simulink model "ANPC_ThreeLevelSPWM_AoultSwitch1_WangJiang"  (Simulink 7.9)
settings: Solver=ode23tb  StartTime=0.0  StopTime=1  MaxStep=1e-4  MinStep=1e-5  RelTol=1e-3
undefined symbols (not defined in the file or in its folder): D1, Delta
libraries: powerlib x101, powerlib_extras x1, simulink x1
settings Model: Creator=xieleisky  LastModifiedBy=H002220
settings SolverCC: InitialStep=1e-5
settings OptimizationCC: InitFltsAndDblsToZero=on
settings DebuggingCC: SaveWithParameterizedLinksMsg=none  SignalResolutionControl=TryResolveAllWithWarning  MultiTaskDSMMsg=warning  MultiTaskCondExecSysMsg=none  StrictBusMsg=Warning
settings RTWCC: IncludeERTFirstTime=on
settings GRTTargetCC: TargetFcnLib=ansi_tfl_tmw.mat  CombineOutputUpdateFcns=off  GRTInterface=on

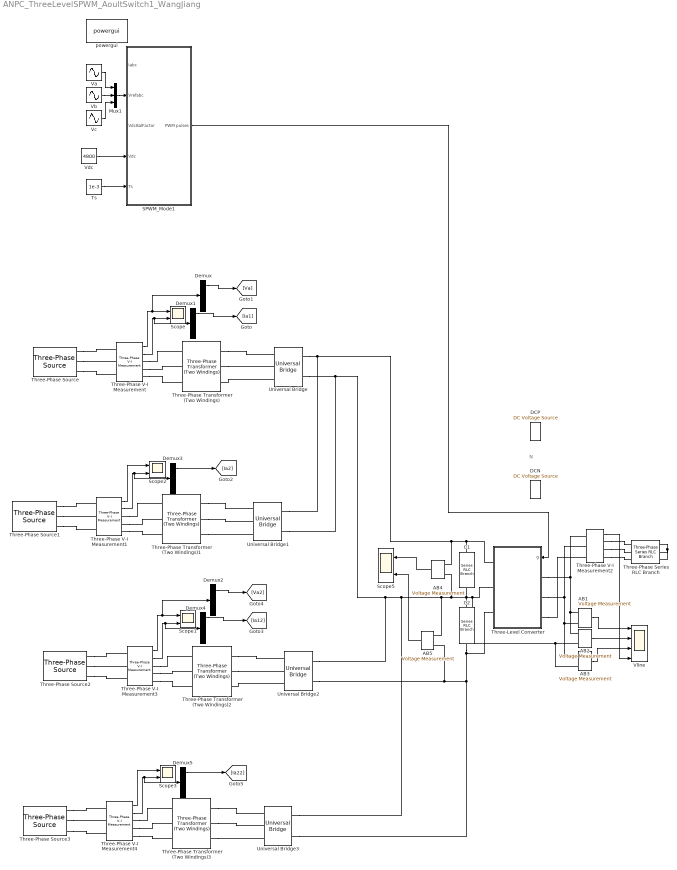
== system ANPC_ThreeLevelSPWM_AoultSwitch1_WangJiang ==
  note: N
  AB{1..5} (5 alike) : powerlib/Measurements/Voltage Measurement  PhasorSimulation=off  OutputType=Complex  PSBequivalent=0
  C1 : powerlib/Elements/Series RLC Branch  LConnTagsString=__new0  RConnTagsString=__new0  BranchType=C  Resistance=1  Inductance=1e-3  SetiL0=off  InitialCurrent=0  Capacitance=8100e-6  Setx0=on  InitialVoltage=2500  Measurements=None
  C2 : powerlib/Elements/Series RLC Branch  LConnTagsString=__new0  RConnTagsString=__new0  BranchType=C  Resistance=1  Inductance=1e-3  SetiL0=off  InitialCurrent=0  Capacitance=8100e-6  Setx0=on  InitialVoltage=2500  Measurements=None
  "DCN " : powerlib/Electrical Sources/DC Voltage Source  Amplitude=300  Measurements=None
  "DCP " : powerlib/Electrical Sources/DC Voltage Source  Amplitude=300  Measurements=None
  Demux{,1..5} (6 alike) : Demux  Outputs=3
  Mux1 : Mux  Inputs=3
  SPWM_Mode1 : Subsystem
  Scope{,1..3,5} (5 alike) : Scope  NumInputPorts=2
      Scope settings: YMin=-5~-5  YMax=5~5
      Scope1 settings: YMin=-5~-5  YMax=5~5  SaveName=ScopeData3
      Scope2 settings: YMin=-5~-5  YMax=5~5  SaveName=ScopeData2
      Scope3 settings: YMin=-5~-5  YMax=5~5  SaveName=ScopeData5
      Scope5 settings: YMin=-5~-5  YMax=5~5  SaveName=ScopeData7
  Three-Level Converter : Subsystem
  Three-Phase Series RLC Branch : powerlib/Elements/Three-Phase Series RLC Branch  LConnTagsString=A|B|C  RConnTagsString=A|B|C  BranchType=RL  Resistance=24.12  Inductance=10.5e-3  Capacitance=1e-6  Measurements=None
  Three-Phase Transformer (Two Windings){,1..3} (4 alike) : powerlib/Elements/Three-Phase Transformer (Two Windings)  Winding1Connection=Delta (D1)  UNITS=pu  NominalPower=[ 1.25e6 , 50 ]  Winding1=[ 25e3 , 0.002 , 0.01 ]  Winding2Connection=Delta (D1)  Winding2=[ 1.8e3 , 0.002 , 0.064 ]  SetSaturation=off  Rm=500  Lm=500  Saturation=[ 0,0 ; 0.0024,1.2 ; 1.0,1.52 ]  Hysteresis=off  DataFile='hysteresis'  SetInitialFlux=off  InitialFluxes=[ 0.8 , -0.8 , 0.7 ]  Measurements=None  MoreParameters=off  BreakLoop=off  DataType=off  TransfoNumber=1
  Three-Phase V-I Measurement{,1,3..4} (4 alike) : powerlib/Measurements/Three-Phase V-I Measurement  VoltageMeasurement=phase-to-phase  SetLabelV=off  LabelV=Vabc  Vpu=off  VpuLL=off  CurrentMeasurement=yes  SetLabelI=off  LabelI=Iabc  Ipu=off  Pbase=100e6  Vbase=500e3  OutputType=Complex  PhasorSimulation=off  PSBequivalent=0
  Three-Phase V-I Measurement2 : powerlib/Measurements/Three-Phase V-I Measurement  VoltageMeasurement=no  SetLabelV=off  LabelV=Vabc  Vpu=off  VpuLL=off  CurrentMeasurement=yes  SetLabelI=off  LabelI=Iabc  Ipu=off  Pbase=100e6  Vbase=500e3  OutputType=Complex  PhasorSimulation=off  PSBequivalent=0
  Three-Phase Source : powerlib/Electrical Sources/Three-Phase Source  Voltage=25e3  PhaseAngle=0  Frequency=50  InternalConnection=Yg  SpecifyImpedance=off  Resistance=1e-5  Inductance=1e-6  ShortCircuitLevel=1e8  BaseVoltage=25e3  XRratio=0.1  BusType=swing  Pref=0  Qref=0  Qmin=-inf  Qmax=inf
  Three-Phase Source1 : powerlib/Electrical Sources/Three-Phase Source  Voltage=25e3  PhaseAngle=15  Frequency=50  InternalConnection=Yg  SpecifyImpedance=off  Resistance=1e-5  Inductance=1e-6  ShortCircuitLevel=1e8  BaseVoltage=25e3  XRratio=0.1  BusType=swing  Pref=0  Qref=0  Qmin=-inf  Qmax=inf
  Three-Phase Source2 : powerlib/Electrical Sources/Three-Phase Source  Voltage=25e3  PhaseAngle=45  Frequency=50  InternalConnection=Yg  SpecifyImpedance=off  Resistance=1e-5  Inductance=1e-6  ShortCircuitLevel=1e8  BaseVoltage=25e3  XRratio=0.1  BusType=swing  Pref=0  Qref=0  Qmin=-inf  Qmax=inf
  Three-Phase Source3 : powerlib/Electrical Sources/Three-Phase Source  Voltage=25e3  PhaseAngle=60  Frequency=50  InternalConnection=Yg  SpecifyImpedance=off  Resistance=1e-5  Inductance=1e-6  ShortCircuitLevel=1e8  BaseVoltage=25e3  XRratio=0.1  BusType=swing  Pref=0  Qref=0  Qmin=-inf  Qmax=inf
  Ts : Constant  Value=1e-3
  Universal Bridge{,1..3} (4 alike) : powerlib/Power Electronics/Universal Bridge  Arms=3  SnubberResistance=1e5  SnubberCapacitance=inf  Device=Diodes  Ron=1e-3  Lon=0  ForwardVoltages="[  0  0  ]"  ForwardVoltage=0.2  GTOparameters=[ 10e-6 , 20e-6 ]  IGBTparameters=[ 1e-6 , 2e-6 ]  Measurements=None  Measurements_2=None  converterType=Rectifier
  Va : Sin  Amplitude=2694  Frequency=100*pi  SampleTime=0
  Vb : Sin  Amplitude=2694  Frequency=100*pi  Phase=-2*pi/3  SampleTime=0
  Vc : Sin  Amplitude=2694  Frequency=100*pi  Phase=2*pi/3  SampleTime=0
  Vdc : Constant  Value=4800
  Vline : Scope  NumInputPorts=4
      settings: TimeRange=0.07315761161915008  YMin=-800~-400~-400~-30  YMax=800~400~400~30  SaveName=A  MaxDataPoints=50000  SampleTime=0.00001
  powergui : powerlib/powergui  SimulationMode=Discrete  SolverType=Tustin  SampleTime=1e-5  frequency=60  SPID=off  DisableSnubberDevices=off  DisableRonSwitches=off  DisableVfSwitches=off  SwTol=0  Interpol=off  DisplayEquations=off  FunctionMessages=off  frequencyindice=0  Pbase=100e6  ErrMax=1e-4  Iterations=50  UnitsV=kV  UnitsW=MW  echomessages=off  HookPort=off  EnableUseOfTLC=off  x0status=blocks  RestoreLinks=warning  ResistiveCurrentMeasurement=off  Frange=[0:2:500]  Ylog=off  Xlog=on  ShowGrid=off  save=off  variable=ZData  structure=ScopeData7  ZoomFFT=off  StartTime=0.2  cycles=1  DisplayStyle=3  fundamental=60  FreqAxis=on  MaxFrequency=3500  frequencyindicesteady=1  RmsSteady=1  display=off  Ts=0  methode=off
  wires:
  Ts/1 -> SPWM_Mode1/5(Ts)
  Vdc/1 -> SPWM_Mode1/4(Vdc)
  AB1/1 -> Vline/1
  AB2/1 -> Vline/2
  AB3/1 -> Vline/3
  Three-Phase V-I Measurement2/1 -> Vline/4
  SPWM_Mode1/1(PWM pulses) -> Three-Level Converter/1(g)
  Mux1/1 -> SPWM_Mode1/2(Vrefabc)
  Vb/1 -> Mux1/2
  Vc/1 -> Mux1/3
  Va/1 -> Mux1/1
  Three-Phase V-I Measurement/2 -> Scope/2, Demux1/1
  Three-Phase V-I Measurement/1 -> Scope/1, Demux/1
  Demux1/1 -> [Ia1]
  Three-Phase V-I Measurement1/2 -> Demux3/1, Scope2/2
  Three-Phase V-I Measurement1/1 -> Scope2/1
  Demux3/1 -> [Ia2]
  Three-Phase V-I Measurement3/2 -> Demux4/1, Scope1/2
  Three-Phase V-I Measurement3/1 -> Demux2/1, Scope1/1
  Demux4/1 -> [Ia12]
  Demux2/1 -> [Va2]
  Three-Phase V-I Measurement4/2 -> Scope3/2, Demux5/1
  Three-Phase V-I Measurement4/1 -> Scope3/1
  Demux5/1 -> [Ia22]
  AB4/1 -> Scope5/1
  AB5/1 -> Scope5/2
  Demux/1 -> [Va]
  connections:
  Three-Level Converter/LConn1 -- AB2/LConn1 -- AB1/LConn1 -- Three-Phase V-I Measurement2/LConn1
  Three-Level Converter/LConn2 -- AB3/LConn1 -- AB1/LConn2 -- Three-Phase V-I Measurement2/LConn2
  Three-Level Converter/LConn3 -- Three-Phase V-I Measurement2/LConn3
  Three-Phase Series RLC Branch/RConn1 -- Three-Phase Series RLC Branch/RConn2 -- Three-Phase Series RLC Branch/RConn3
  Three-Phase V-I Measurement2/RConn1 -- Three-Phase Series RLC Branch/LConn1
  Three-Phase V-I Measurement2/RConn2 -- Three-Phase Series RLC Branch/LConn2
  Three-Phase V-I Measurement2/RConn3 -- Three-Phase Series RLC Branch/LConn3
  Three-Phase V-I Measurement/RConn3 -- Three-Phase Transformer (Two Windings)/LConn3
  Three-Phase Source1/RConn2 -- Three-Phase V-I Measurement1/LConn2
  Three-Phase Source1/RConn3 -- Three-Phase V-I Measurement1/LConn3
  Three-Phase V-I Measurement1/RConn1 -- Three-Phase Transformer (Two Windings)1/LConn1
  Three-Phase Transformer (Two Windings)1/RConn1 -- Universal Bridge1/LConn1
  Three-Phase V-I Measurement1/RConn3 -- Three-Phase Transformer (Two Windings)1/LConn3
  Three-Phase Source/RConn3 -- Three-Phase V-I Measurement/LConn3
  Three-Phase Transformer (Two Windings)/RConn3 -- Universal Bridge/LConn3
  Three-Phase Source1/RConn1 -- Three-Phase V-I Measurement1/LConn1
  Three-Phase V-I Measurement/RConn1 -- Three-Phase Transformer (Two Windings)/LConn1
  Three-Phase Transformer (Two Windings)1/RConn2 -- Universal Bridge1/LConn2
  Three-Phase V-I Measurement/RConn2 -- Three-Phase Transformer (Two Windings)/LConn2
  Three-Phase Transformer (Two Windings)/RConn1 -- Universal Bridge/LConn1
  Three-Phase Source/RConn1 -- Three-Phase V-I Measurement/LConn1
  Three-Phase Source/RConn2 -- Three-Phase V-I Measurement/LConn2
  Three-Phase Transformer (Two Windings)/RConn2 -- Universal Bridge/LConn2
  Three-Phase V-I Measurement1/RConn2 -- Three-Phase Transformer (Two Windings)1/LConn2
  Three-Phase Transformer (Two Windings)1/RConn3 -- Universal Bridge1/LConn3
  Universal Bridge2/RConn2 -- C2/RConn1 -- Three-Level Converter/RConn3 -- Universal Bridge3/RConn2 -- AB5/LConn2
  Universal Bridge/RConn1 -- Universal Bridge1/RConn1 -- Three-Level Converter/RConn1 -- C1/LConn1 -- AB4/LConn1
  C1/RConn1 -- C2/LConn1 -- Three-Level Converter/RConn2 -- AB4/LConn2 -- Universal Bridge/RConn2 -- Universal Bridge1/RConn2 -- Universal Bridge2/RConn1 -- Universal Bridge3/RConn1 -- AB5/LConn1 -- AB2/LConn2 -- AB3/LConn2
  Three-Phase Source2/RConn1 -- Three-Phase V-I Measurement3/LConn1
  Three-Phase Source2/RConn3 -- Three-Phase V-I Measurement3/LConn3
  Three-Phase Transformer (Two Windings)3/RConn1 -- Universal Bridge3/LConn1
  Three-Phase Transformer (Two Windings)3/RConn2 -- Universal Bridge3/LConn2
  Three-Phase Source3/RConn3 -- Three-Phase V-I Measurement4/LConn3
  Three-Phase Source3/RConn2 -- Three-Phase V-I Measurement4/LConn2
  Three-Phase Transformer (Two Windings)2/RConn2 -- Universal Bridge2/LConn2
  Three-Phase Transformer (Two Windings)3/RConn3 -- Universal Bridge3/LConn3
  Three-Phase Source2/RConn2 -- Three-Phase V-I Measurement3/LConn2
  Three-Phase V-I Measurement4/RConn1 -- Three-Phase Transformer (Two Windings)3/LConn1
  Three-Phase V-I Measurement4/RConn2 -- Three-Phase Transformer (Two Windings)3/LConn2
  Three-Phase Transformer (Two Windings)2/RConn1 -- Universal Bridge2/LConn1
  Three-Phase Source3/RConn1 -- Three-Phase V-I Measurement4/LConn1
  Three-Phase V-I Measurement3/RConn1 -- Three-Phase Transformer (Two Windings)2/LConn1
  Three-Phase Transformer (Two Windings)2/RConn3 -- Universal Bridge2/LConn3
  Three-Phase V-I Measurement3/RConn3 -- Three-Phase Transformer (Two Windings)2/LConn3
  Three-Phase V-I Measurement4/RConn3 -- Three-Phase Transformer (Two Windings)3/LConn3
  Three-Phase V-I Measurement3/RConn2 -- Three-Phase Transformer (Two Windings)2/LConn2

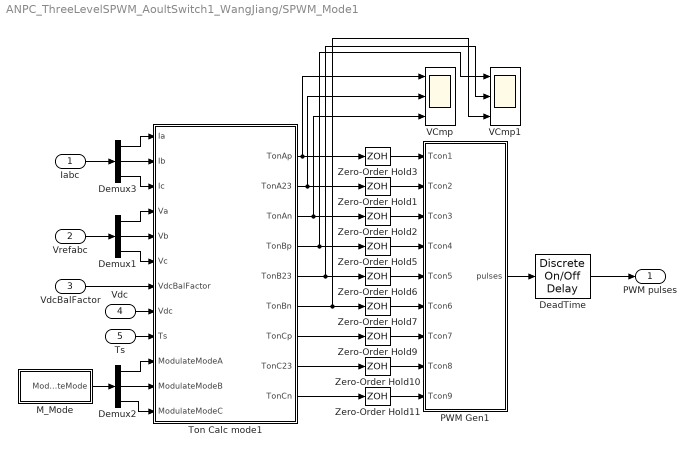
== system ANPC_ThreeLevelSPWM_AoultSwitch1_WangJiang/SPWM_Mode1 ==
  Iabc : Inport
  Vrefabc : Inport  Port=2
  VdcBalFactor : Inport  Port=3
  Vdc : Inport  Port=4
  Ts : Inport  Port=5
  DeadTime : powerlib_extras/Discrete  Control Blocks/Discrete On//Off Delay  type_delay=On delay  delay=20e-6  ic=4e-5  Ts=1e-5
  Demux1 : Demux  Outputs=3
  Demux2 : Demux  Outputs=3
  Demux3 : Demux  Outputs=3
  M_Mode : Subsystem
  PWM Gen1 : Subsystem
  Ton Calc mode1 : MATLAB Function  TreatAsAtomicUnit=on
  VCmp : Scope  NumInputPorts=3
      settings: TimeRange=0.5  YMin=0.00015~0~0.00065  YMax=0.00035~0.001~0.00085  SaveName=A3  MaxDataPoints=50000  SampleTime=0.00001
  VCmp1 : Scope  NumInputPorts=3
      settings: TimeRange=0.05095198250172486  YMin=0~0~0  YMax=0.001~0.001~0.001  SaveName=A1  MaxDataPoints=50000  SampleTime=0.00001
  Zero-Order Hold{1..3,5..7,9..11} (9 alike) : ZeroOrderHold  SampleTime=1/1500
  PWM pulses : Outport
  wires:
  Demux1/2 -> Ton Calc mode1/5(Vb)
  Demux1/3 -> Ton Calc mode1/6(Vc)
  Vdc/1 -> Ton Calc mode1/8(Vdc)
  Ts/1 -> Ton Calc mode1/9(Ts)
  Zero-Order Hold3/1 -> PWM Gen1/1(Tcon1)
  Zero-Order Hold2/1 -> PWM Gen1/3(Tcon3)
  Zero-Order Hold11/1 -> PWM Gen1/9(Tcon9)
  PWM Gen1/1(pulses) -> DeadTime/1
  Zero-Order Hold10/1 -> PWM Gen1/8(Tcon8)
  Zero-Order Hold9/1 -> PWM Gen1/7(Tcon7)
  Zero-Order Hold7/1 -> PWM Gen1/6(Tcon6)
  Zero-Order Hold6/1 -> PWM Gen1/5(Tcon5)
  Zero-Order Hold5/1 -> PWM Gen1/4(Tcon4)
  Zero-Order Hold1/1 -> PWM Gen1/2(Tcon2)
  Ton Calc mode1/1(TonAp) -> VCmp/1, Zero-Order Hold3/1
  Ton Calc mode1/2(TonA23) -> VCmp/2, Zero-Order Hold1/1
  Ton Calc mode1/3(TonAn) -> VCmp/3, Zero-Order Hold2/1
  Ton Calc mode1/4(TonBp) -> VCmp1/1, Zero-Order Hold5/1
  Ton Calc mode1/5(TonB23) -> VCmp1/2, Zero-Order Hold6/1
  Ton Calc mode1/6(TonBn) -> VCmp1/3, Zero-Order Hold7/1
  Ton Calc mode1/7(TonCp) -> Zero-Order Hold9/1
  Ton Calc mode1/8(TonC23) -> Zero-Order Hold10/1
  Ton Calc mode1/9(TonCn) -> Zero-Order Hold11/1
  Demux3/1 -> Ton Calc mode1/1(Ia)
  Demux3/2 -> Ton Calc mode1/2(Ib)
  Demux3/3 -> Ton Calc mode1/3(Ic)
  Iabc/1 -> Demux3/1
  Demux1/1 -> Ton Calc mode1/4(Va)
  Vrefabc/1 -> Demux1/1
  Demux2/2 -> Ton Calc mode1/11(ModulateModeB)
  Demux2/3 -> Ton Calc mode1/12(ModulateModeC)
  Demux2/1 -> Ton Calc mode1/10(ModulateModeA)
  VdcBalFactor/1 -> Ton Calc mode1/7(VdcBalFactor)
  M_Mode/1(ModulateMode) -> Demux2/1
  DeadTime/1 -> PWM pulses/1

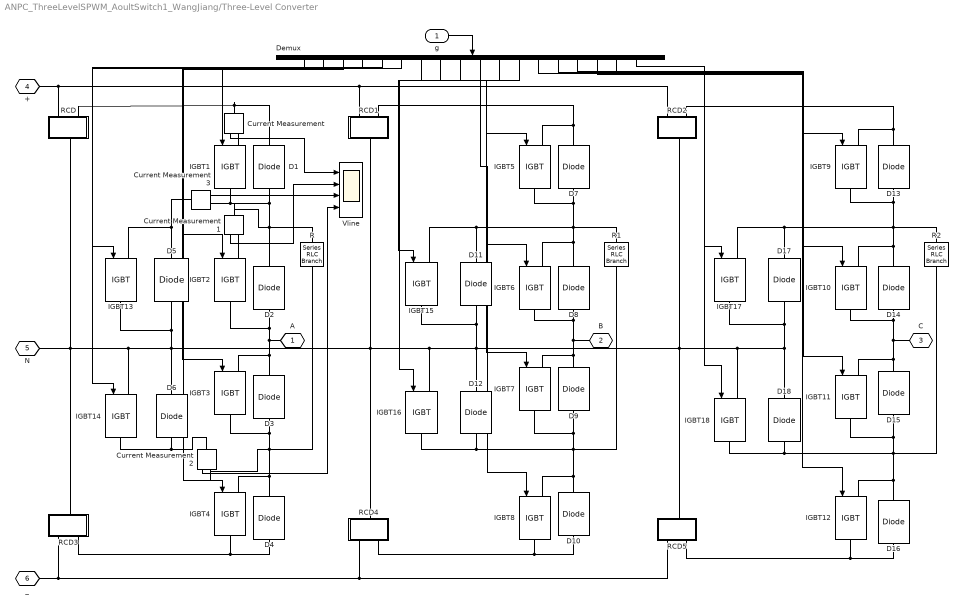
== system ANPC_ThreeLevelSPWM_AoultSwitch1_WangJiang/Three-Level Converter ==
  g : Inport
  Current Measurement{,1..3} (4 alike) : powerlib/Measurements/Current Measurement  PhasorSimulation=off  OutputType=Complex  PSBequivalent=0
  D{1..18} (18 alike) : powerlib/Power Electronics/Diode  Ron=1e-3  Lon=0  Vf=0.8  IC=0  UseSnubber=off  Rs=inf  Cs=0  Measurements=off
  Demux : Demux  Outputs=18
  IGBT{1..18} (18 alike) : powerlib/Power Electronics/IGBT  Ron=1e-3  Lon=0  Vf=1  Tf=0  Tt=0  IC=0  Rs=1e5  Cs=inf  Measurements=off
  R : powerlib/Elements/Series RLC Branch  LConnTagsString=__new0  RConnTagsString=__new0  BranchType=R  Resistance=44000  Inductance=1.0  SetiL0=off  InitialCurrent=0  Capacitance=1.0  Setx0=off  InitialVoltage=0  Measurements=None
  R1 : powerlib/Elements/Series RLC Branch  LConnTagsString=__new0  RConnTagsString=__new0  BranchType=R  Resistance=44000  Inductance=1.0  SetiL0=off  InitialCurrent=0  Capacitance=1.0  Setx0=off  InitialVoltage=0  Measurements=None
  R2 : powerlib/Elements/Series RLC Branch  LConnTagsString=__new0  RConnTagsString=__new0  BranchType=R  Resistance=44000  Inductance=1.0  SetiL0=off  InitialCurrent=0  Capacitance=1.0  Setx0=off  InitialVoltage=0  Measurements=None
  RCD : Subsystem
  RCD1 : Subsystem
  RCD2 : Subsystem
  RCD3 : Subsystem
  RCD4 : Subsystem
  RCD5 : Subsystem
  Vline : Scope  NumInputPorts=4
      settings: TimeRange=0.05095198250172486  YMin=-10~-10~-30~-35  YMax=40~40~30~35  SaveName=A2  MaxDataPoints=50000  SampleTime=0.00001
  A : PMIOPort  Tag=PMCPort  Port=1  Side=Left
  B : PMIOPort  Tag=PMCPort  Port=2  Side=Left
  C : PMIOPort  Tag=PMCPort  Port=3  Side=Left
  + : PMIOPort  Tag=PMCPort  Port=4  Side=Right
  N : PMIOPort  Tag=PMCPort  Port=5  Side=Right
  _ : PMIOPort  Tag=PMCPort  Port=6  Side=Right
  wires:
  g/1 -> Demux/1
  Demux/1 -> IGBT1/1
  Demux/2 -> IGBT2/1
  Demux/3 -> IGBT3/1
  Demux/4 -> IGBT4/1
  Demux/5 -> IGBT13/1
  Demux/6 -> IGBT14/1
  Demux/7 -> IGBT5/1
  Demux/8 -> IGBT6/1
  Demux/9 -> IGBT7/1
  Demux/10 -> IGBT8/1
  Demux/11 -> IGBT15/1
  Demux/12 -> IGBT16/1
  Demux/13 -> IGBT9/1
  Demux/14 -> IGBT10/1
  Demux/15 -> IGBT11/1
  Demux/16 -> IGBT12/1
  Demux/17 -> IGBT17/1
  Demux/18 -> IGBT18/1
  Current Measurement/1 -> Vline/1
  Current Measurement1/1 -> Vline/2
  Current Measurement3/1 -> Vline/3
  Current Measurement2/1 -> Vline/4
  connections:
  R/LConn1 -- Current Measurement1/LConn1 -- D2/RConn1 -- IGBT1/RConn1 -- Current Measurement3/RConn1 -- D1/LConn1
  IGBT4/LConn1 -- D4/RConn1 -- Current Measurement2/RConn1 -- R/RConn1 -- D3/LConn1 -- IGBT3/RConn1
  IGBT8/LConn1 -- D10/RConn1 -- IGBT7/RConn1 -- D9/LConn1 -- IGBT16/RConn1 -- D12/LConn1 -- R1/RConn1
  IGBT10/LConn1 -- D14/RConn1 -- D13/LConn1 -- IGBT9/RConn1 -- D17/RConn1 -- IGBT17/LConn1 -- R2/LConn1
  IGBT10/RConn1 -- IGBT11/LConn1 -- D15/RConn1 -- C/RConn1 -- D14/LConn1
  IGBT11/RConn1 -- D15/LConn1 -- IGBT18/RConn1 -- D18/LConn1 -- D16/RConn1 -- IGBT12/LConn1 -- R2/RConn1
  D12/RConn1 -- RCD5/RConn1 -- RCD2/RConn1 -- IGBT18/LConn1 -- IGBT17/RConn1 -- D17/LConn1 -- D18/RConn1 -- IGBT16/LConn1 -- D6/RConn1 -- IGBT14/LConn1 -- RCD/RConn1 -- N/RConn1 -- RCD3/RConn1 -- IGBT13/RConn1 -- D5/LConn1 -- RCD4/RConn1 -- RCD1/RConn1 -- IGBT15/RConn1 -- D11/LConn1
  RCD/LConn2 -- Current Measurement/LConn1 -- D1/RConn1
  RCD2/LConn1 -- RCD/LConn1 -- +/RConn1 -- RCD1/LConn1
  R1/LConn1 -- IGBT15/LConn1 -- D11/RConn1 -- D7/LConn1 -- IGBT5/RConn1 -- IGBT6/LConn1 -- D8/RConn1
  D3/RConn1 -- IGBT3/LConn1 -- IGBT2/RConn1 -- D2/LConn1 -- A/RConn1
  D7/RConn1 -- IGBT5/LConn1 -- RCD1/LConn2
  IGBT9/LConn1 -- RCD2/LConn2 -- D13/RConn1
  D4/LConn1 -- RCD3/LConn2 -- IGBT4/RConn1
  D10/LConn1 -- RCD4/LConn2 -- IGBT8/RConn1
  RCD3/LConn1 -- _/RConn1 -- RCD5/LConn1 -- RCD4/LConn1
  D16/LConn1 -- RCD5/LConn2 -- IGBT12/RConn1
  IGBT7/LConn1 -- D8/LConn1 -- IGBT6/RConn1 -- B/RConn1 -- D9/RConn1
  Current Measurement/RConn1 -- IGBT1/LConn1
  Current Measurement1/RConn1 -- IGBT2/LConn1
  IGBT14/RConn1 -- Current Measurement2/LConn1 -- D6/LConn1
  IGBT13/LConn1 -- Current Measurement3/LConn1 -- D5/RConn1

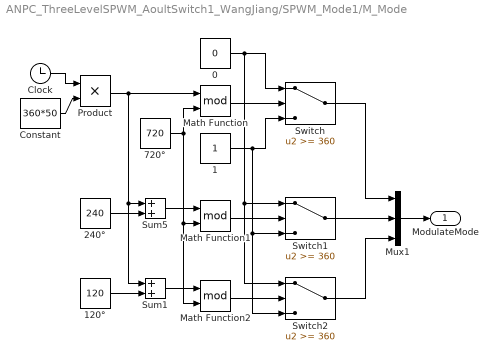
== system ANPC_ThreeLevelSPWM_AoultSwitch1_WangJiang/SPWM_Mode1/M_Mode ==
  0 : Constant  Value=0
  1 : Constant
  120° : Constant  Value=120
  240° : Constant  Value=240
  720° : Constant  Value=720
  Clock : Clock
  Constant : Constant  Value=360*50
  Math Function : Math  Operator=mod  SaturateOnIntegerOverflow=on
  Math Function1 : Math  Operator=mod  SaturateOnIntegerOverflow=on
  Math Function2 : Math  Operator=mod  SaturateOnIntegerOverflow=on
  Mux1 : Mux  Inputs=3
  Product : Product  RndMeth=Zero
  Sum1 : Sum  SaturateOnIntegerOverflow=on  InputSameDT=on  OutDataTypeStr=Inherit: Same as first input
  Sum5 : Sum  SaturateOnIntegerOverflow=on  InputSameDT=on  OutDataTypeStr=Inherit: Same as first input
  Switch : Switch  Threshold=360
  Switch1 : Switch  Threshold=360
  Switch2 : Switch  Threshold=360
  ModulateMode : Outport
  wires:
  Constant/1 -> Product/2
  Clock/1 -> Product/1
  Sum5/1 -> Math Function1/1
  Product/1 -> Sum1/1, Sum5/1, Math Function/1
  Sum1/1 -> Math Function2/1
  720°/1 -> Math Function/2, Math Function2/2, Math Function1/2
  240°/1 -> Sum5/2
  120°/1 -> Sum1/2
  Mux1/1 -> ModulateMode/1
  Math Function/1 -> Switch/2
  Math Function1/1 -> Switch1/2
  Math Function2/1 -> Switch2/2
  1/1 -> Switch/3, Switch2/3, Switch1/3
  0/1 -> Switch2/1, Switch1/1, Switch/1
  Switch/1 -> Mux1/1
  Switch1/1 -> Mux1/2
  Switch2/1 -> Mux1/3

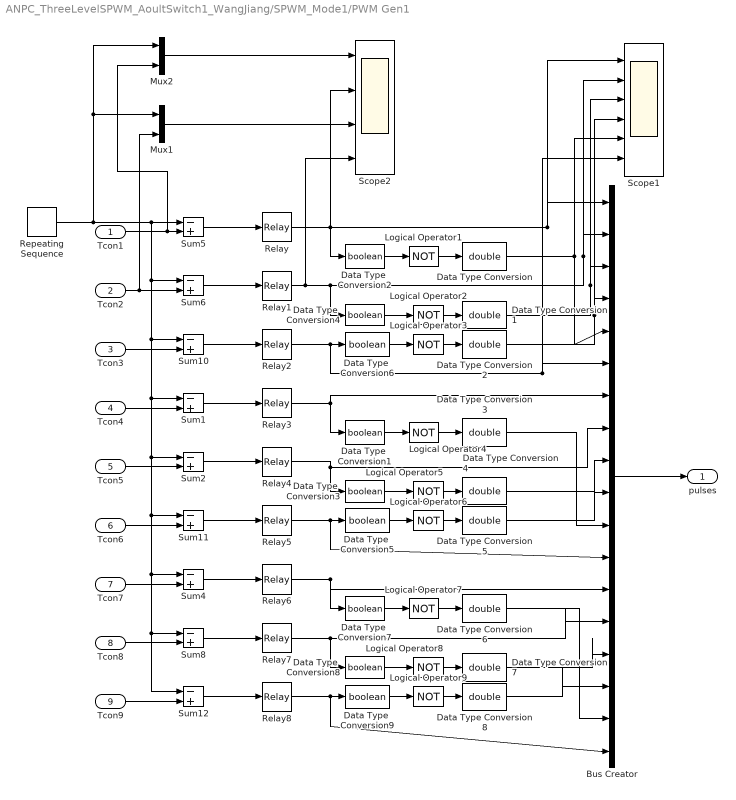
== system ANPC_ThreeLevelSPWM_AoultSwitch1_WangJiang/SPWM_Mode1/PWM Gen1 ==
  Tcon1 : Inport
  Tcon2 : Inport  Port=2
  Tcon3 : Inport  Port=3
  Tcon4 : Inport  Port=4
  Tcon5 : Inport  Port=5
  Tcon6 : Inport  Port=6
  Tcon7 : Inport  Port=7
  Tcon8 : Inport  Port=8
  Tcon9 : Inport  Port=9
  Bus Creator : BusCreator  Inputs=18
  Data Type  Conversion{1..9} (9 alike) : DataTypeConversion  OutDataTypeStr=boolean  SaturateOnIntegerOverflow=on  RndMeth=Zero
  Data Type Conversion{,1..8} (9 alike) : DataTypeConversion  OutDataTypeStr=double
  Logical Operator{1..9} (9 alike) : Logic  Operator=NOT
  Mux1 : Mux  Inputs=2
  Mux2 : Mux  Inputs=2
  Relay{,1..8} (9 alike) : Relay  OnSwitchValue=1e-6  OffSwitchValue=-1e-6
  Repeating Sequence : simulink/Sources/Repeating Sequence  rep_seq_t=[0 1/1500 1/750]  rep_seq_y=[1e-3 0 1e-3]
  Scope1 : Scope  NumInputPorts=6
      settings: YMin=-0.5~-0.5~-0.5~-0.5~-0.5~-0.5  YMax=1.5~1.5~1.5~1.5~1.5~1.5  SaveName=ScopeData4  MaxDataPoints=10000
  Scope2 : Scope  NumInputPorts=4
      settings: YMin=-0.5~-0.5~-0.5~-0.5  YMax=1.5~1.5~1.5~1.5  MaxDataPoints=10000
  Sum{1..2,4..6,8,10..12} (9 alike) : Sum  Inputs=-+  SaturateOnIntegerOverflow=on  InputSameDT=on  OutDataTypeStr=Inherit: Same as first input
  pulses : Outport
  wires:
  Bus Creator/1 -> pulses/1
  Tcon1/1 -> Mux2/2, Sum5/2
  Tcon2/1 -> Mux1/2, Sum6/2
  Sum5/1 -> Relay/1
  Relay/1 -> Bus Creator/1, Scope1/1, Scope2/2, Data Type  Conversion2/1
  Sum6/1 -> Relay1/1
  Relay1/1 -> Scope2/4, Data Type  Conversion4/1, Bus Creator/2, Scope1/2
  Relay2/1 -> Bus Creator/6, Scope1/6, Data Type  Conversion6/1
  Logical Operator1/1 -> Data Type Conversion/1
  Data Type  Conversion2/1 -> Logical Operator1/1
  Logical Operator2/1 -> Data Type Conversion1/1
  Data Type  Conversion4/1 -> Logical Operator2/1
  Logical Operator3/1 -> Data Type Conversion2/1
  Data Type  Conversion6/1 -> Logical Operator3/1
  Tcon4/1 -> Sum1/2
  Tcon5/1 -> Sum2/2
  Sum1/1 -> Relay3/1
  Relay3/1 -> Data Type  Conversion1/1, Bus Creator/7
  Sum2/1 -> Relay4/1
  Relay4/1 -> Data Type  Conversion3/1, Bus Creator/8
  Relay5/1 -> Bus Creator/12, Data Type  Conversion5/1
  Logical Operator4/1 -> Data Type Conversion3/1
  Data Type  Conversion1/1 -> Logical Operator4/1
  Logical Operator5/1 -> Data Type Conversion4/1
  Data Type  Conversion3/1 -> Logical Operator5/1
  Logical Operator6/1 -> Data Type Conversion5/1
  Data Type  Conversion5/1 -> Logical Operator6/1
  Data Type Conversion/1 -> Bus Creator/5, Scope1/5
  Data Type Conversion1/1 -> Bus Creator/3, Scope1/3
  Data Type Conversion2/1 -> Bus Creator/4, Scope1/4
  Tcon7/1 -> Sum4/2
  Tcon8/1 -> Sum8/2
  Tcon9/1 -> Sum12/2
  Sum4/1 -> Relay6/1
  Relay6/1 -> Data Type  Conversion7/1, Bus Creator/13
  Sum8/1 -> Relay7/1
  Relay7/1 -> Bus Creator/14, Data Type  Conversion8/1
  Relay8/1 -> Bus Creator/18, Data Type  Conversion9/1
  Logical Operator7/1 -> Data Type Conversion6/1
  Data Type  Conversion7/1 -> Logical Operator7/1
  Logical Operator8/1 -> Data Type Conversion7/1
  Data Type  Conversion8/1 -> Logical Operator8/1
  Logical Operator9/1 -> Data Type Conversion8/1
  Data Type  Conversion9/1 -> Logical Operator9/1
  Data Type Conversion3/1 -> Bus Creator/11
  Data Type Conversion4/1 -> Bus Creator/9
  Data Type Conversion5/1 -> Bus Creator/10
  Data Type Conversion6/1 -> Bus Creator/17
  Data Type Conversion7/1 -> Bus Creator/15
  Data Type Conversion8/1 -> Bus Creator/16
  Sum10/1 -> Relay2/1
  Sum11/1 -> Relay5/1
  Sum12/1 -> Relay8/1
  Tcon3/1 -> Sum10/2
  Tcon6/1 -> Sum11/2
  Mux2/1 -> Scope2/1
  Mux1/1 -> Scope2/3
  Repeating Sequence/1 -> Mux1/1, Mux2/1, Sum2/1, Sum11/1, Sum12/1, Sum8/1, Sum4/1, Sum1/1, Sum10/1, Sum6/1, Sum5/1

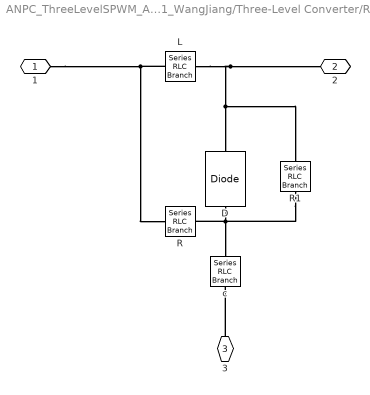
== system ANPC_ThreeLevelSPWM_AoultSwitch1_WangJiang/Three-Level Converter/RCD ==
  D : powerlib/Power Electronics/Diode  Ron=1e-3  Lon=0  Vf=0.8  IC=0  UseSnubber=off  Rs=inf  Cs=0  Measurements=off
  L : powerlib/Elements/Series RLC Branch  LConnTagsString=__new0  RConnTagsString=__new0  BranchType=RL  Resistance=1e-4  Inductance=5.59e-6  SetiL0=off  InitialCurrent=0  Capacitance=1.0  Setx0=off  InitialVoltage=0  Measurements=None
  R : powerlib/Elements/Series RLC Branch  LConnTagsString=__new0  RConnTagsString=__new0  BranchType=R  Resistance=0.5  Inductance=1.0  SetiL0=off  InitialCurrent=0  Capacitance=1.0  Setx0=off  InitialVoltage=0  Measurements=None
  R1 : powerlib/Elements/Series RLC Branch  LConnTagsString=__new0  RConnTagsString=__new0  BranchType=R  Resistance=1e6  Inductance=1.0  SetiL0=off  InitialCurrent=0  Capacitance=1.0  Setx0=off  InitialVoltage=0  Measurements=None
  c : powerlib/Elements/Series RLC Branch  LConnTagsString=__new0  RConnTagsString=__new0  BranchType=C  Resistance=1  Inductance=1.0  SetiL0=off  InitialCurrent=0  Capacitance=5e-6  Setx0=off  InitialVoltage=0  Measurements=None
  1 : PMIOPort  Port=1  Side=Left
  2 : PMIOPort  Port=2  Side=Left
  3 : PMIOPort  Port=3  Side=Right
  connections:
  L/RConn1 -- 2/RConn1 -- D/LConn1 -- R1/LConn1
  D/RConn1 -- R/RConn1 -- c/LConn1 -- R1/RConn1
  L/LConn1 -- R/LConn1 -- 1/RConn1
  3/RConn1 -- c/RConn1

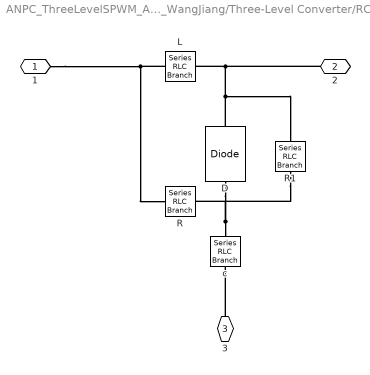
== system ANPC_ThreeLevelSPWM_AoultSwitch1_WangJiang/Three-Level Converter/RCD1 ==
  D : powerlib/Power Electronics/Diode  Ron=1e-3  Lon=0  Vf=0.8  IC=0  UseSnubber=off  Rs=inf  Cs=0  Measurements=off
  L : powerlib/Elements/Series RLC Branch  LConnTagsString=__new0  RConnTagsString=__new0  BranchType=RL  Resistance=1e-4  Inductance=5.59e-6  SetiL0=off  InitialCurrent=0  Capacitance=1.0  Setx0=off  InitialVoltage=0  Measurements=None
  R : powerlib/Elements/Series RLC Branch  LConnTagsString=__new0  RConnTagsString=__new0  BranchType=R  Resistance=0.5  Inductance=1.0  SetiL0=off  InitialCurrent=0  Capacitance=1.0  Setx0=off  InitialVoltage=0  Measurements=None
  R1 : powerlib/Elements/Series RLC Branch  LConnTagsString=__new0  RConnTagsString=__new0  BranchType=R  Resistance=1e6  Inductance=1.0  SetiL0=off  InitialCurrent=0  Capacitance=1.0  Setx0=off  InitialVoltage=0  Measurements=None
  c : powerlib/Elements/Series RLC Branch  LConnTagsString=__new0  RConnTagsString=__new0  BranchType=C  Resistance=1  Inductance=1.0  SetiL0=off  InitialCurrent=0  Capacitance=5e-6  Setx0=off  InitialVoltage=0  Measurements=None
  1 : PMIOPort  Port=1  Side=Left
  2 : PMIOPort  Port=2  Side=Left
  3 : PMIOPort  Port=3  Side=Right
  connections:
  3/RConn1 -- c/RConn1
  1/RConn1 -- R/LConn1 -- L/LConn1
  c/LConn1 -- R/RConn1 -- D/RConn1 -- R1/RConn1
  D/LConn1 -- L/RConn1 -- 2/RConn1 -- R1/LConn1

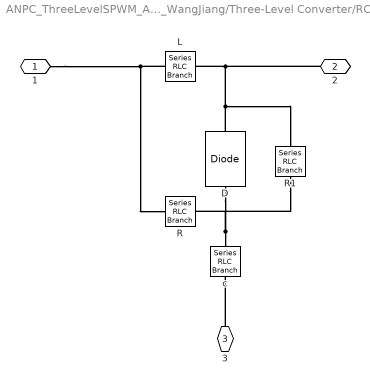
== system ANPC_ThreeLevelSPWM_AoultSwitch1_WangJiang/Three-Level Converter/RCD2 ==
  D : powerlib/Power Electronics/Diode  Ron=1e-3  Lon=0  Vf=0.8  IC=0  UseSnubber=off  Rs=inf  Cs=0  Measurements=off
  L : powerlib/Elements/Series RLC Branch  LConnTagsString=__new0  RConnTagsString=__new0  BranchType=L  Resistance=500^2/200e3  Inductance=5.59e-6  SetiL0=off  InitialCurrent=0  Capacitance=1.0  Setx0=off  InitialVoltage=0  Measurements=None
  R : powerlib/Elements/Series RLC Branch  LConnTagsString=__new0  RConnTagsString=__new0  BranchType=R  Resistance=0.5  Inductance=1.0  SetiL0=off  InitialCurrent=0  Capacitance=1.0  Setx0=off  InitialVoltage=0  Measurements=None
  R1 : powerlib/Elements/Series RLC Branch  LConnTagsString=__new0  RConnTagsString=__new0  BranchType=R  Resistance=1e6  Inductance=1.0  SetiL0=off  InitialCurrent=0  Capacitance=1.0  Setx0=off  InitialVoltage=0  Measurements=None
  c : powerlib/Elements/Series RLC Branch  LConnTagsString=__new0  RConnTagsString=__new0  BranchType=C  Resistance=1  Inductance=1.0  SetiL0=off  InitialCurrent=0  Capacitance=5e-6  Setx0=off  InitialVoltage=0  Measurements=None
  1 : PMIOPort  Port=1  Side=Left
  2 : PMIOPort  Port=2  Side=Left
  3 : PMIOPort  Port=3  Side=Right
  connections:
  3/RConn1 -- c/RConn1
  1/RConn1 -- R/LConn1 -- L/LConn1
  c/LConn1 -- R/RConn1 -- D/RConn1 -- R1/RConn1
  D/LConn1 -- L/RConn1 -- 2/RConn1 -- R1/LConn1

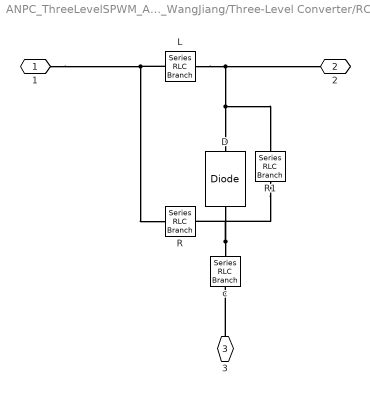
== system ANPC_ThreeLevelSPWM_AoultSwitch1_WangJiang/Three-Level Converter/RCD3 ==
  D : powerlib/Power Electronics/Diode  Ron=1e-3  Lon=0  Vf=0.8  IC=0  UseSnubber=off  Rs=inf  Cs=0  Measurements=off
  L : powerlib/Elements/Series RLC Branch  LConnTagsString=__new0  RConnTagsString=__new0  BranchType=RL  Resistance=1e-4  Inductance=5.59e-6  SetiL0=off  InitialCurrent=0  Capacitance=1.0  Setx0=off  InitialVoltage=0  Measurements=None
  R : powerlib/Elements/Series RLC Branch  LConnTagsString=__new0  RConnTagsString=__new0  BranchType=R  Resistance=0.5  Inductance=1.0  SetiL0=off  InitialCurrent=0  Capacitance=1.0  Setx0=off  InitialVoltage=0  Measurements=None
  R1 : powerlib/Elements/Series RLC Branch  LConnTagsString=__new0  RConnTagsString=__new0  BranchType=R  Resistance=1e6  Inductance=1.0  SetiL0=off  InitialCurrent=0  Capacitance=1.0  Setx0=off  InitialVoltage=0  Measurements=None
  c : powerlib/Elements/Series RLC Branch  LConnTagsString=__new0  RConnTagsString=__new0  BranchType=C  Resistance=1  Inductance=1.0  SetiL0=off  InitialCurrent=0  Capacitance=5e-6  Setx0=off  InitialVoltage=0  Measurements=None
  1 : PMIOPort  Port=1  Side=Left
  2 : PMIOPort  Port=2  Side=Left
  3 : PMIOPort  Port=3  Side=Right
  connections:
  3/RConn1 -- c/RConn1
  1/RConn1 -- R/LConn1 -- L/LConn1
  c/LConn1 -- R/RConn1 -- D/RConn1 -- R1/RConn1
  L/RConn1 -- 2/RConn1 -- D/LConn1 -- R1/LConn1

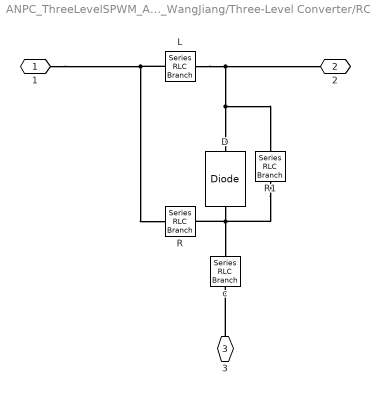
== system ANPC_ThreeLevelSPWM_AoultSwitch1_WangJiang/Three-Level Converter/RCD4 ==
  D : powerlib/Power Electronics/Diode  Ron=1e-3  Lon=0  Vf=0.8  IC=0  UseSnubber=off  Rs=inf  Cs=0  Measurements=off
  L : powerlib/Elements/Series RLC Branch  LConnTagsString=__new0  RConnTagsString=__new0  BranchType=RL  Resistance=1e-4  Inductance=5.59e-6  SetiL0=off  InitialCurrent=0  Capacitance=1.0  Setx0=off  InitialVoltage=0  Measurements=None
  R : powerlib/Elements/Series RLC Branch  LConnTagsString=__new0  RConnTagsString=__new0  BranchType=R  Resistance=0.5  Inductance=1.0  SetiL0=off  InitialCurrent=0  Capacitance=1.0  Setx0=off  InitialVoltage=0  Measurements=None
  R1 : powerlib/Elements/Series RLC Branch  LConnTagsString=__new0  RConnTagsString=__new0  BranchType=R  Resistance=1e6  Inductance=1.0  SetiL0=off  InitialCurrent=0  Capacitance=1.0  Setx0=off  InitialVoltage=0  Measurements=None
  c : powerlib/Elements/Series RLC Branch  LConnTagsString=__new0  RConnTagsString=__new0  BranchType=C  Resistance=1  Inductance=1.0  SetiL0=off  InitialCurrent=0  Capacitance=5e-6  Setx0=off  InitialVoltage=0  Measurements=None
  1 : PMIOPort  Port=1  Side=Left
  2 : PMIOPort  Port=2  Side=Left
  3 : PMIOPort  Port=3  Side=Right
  connections:
  L/RConn1 -- R1/LConn1 -- D/LConn1 -- 2/RConn1
  R1/RConn1 -- D/RConn1 -- R/RConn1 -- c/LConn1
  L/LConn1 -- R/LConn1 -- 1/RConn1
  3/RConn1 -- c/RConn1

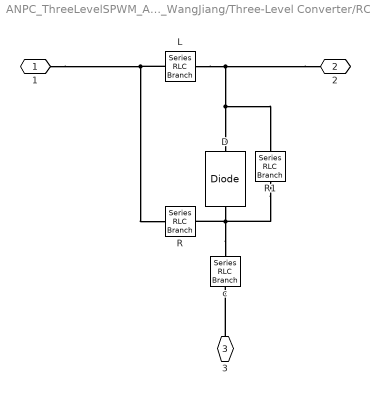
== system ANPC_ThreeLevelSPWM_AoultSwitch1_WangJiang/Three-Level Converter/RCD5 ==
  D : powerlib/Power Electronics/Diode  Ron=1e-3  Lon=0  Vf=0.8  IC=0  UseSnubber=off  Rs=inf  Cs=0  Measurements=off
  L : powerlib/Elements/Series RLC Branch  LConnTagsString=__new0  RConnTagsString=__new0  BranchType=RL  Resistance=1e-4  Inductance=5.59e-6  SetiL0=off  InitialCurrent=0  Capacitance=1.0  Setx0=off  InitialVoltage=0  Measurements=None
  R : powerlib/Elements/Series RLC Branch  LConnTagsString=__new0  RConnTagsString=__new0  BranchType=R  Resistance=0.5  Inductance=1.0  SetiL0=off  InitialCurrent=0  Capacitance=1.0  Setx0=off  InitialVoltage=0  Measurements=None
  R1 : powerlib/Elements/Series RLC Branch  LConnTagsString=__new0  RConnTagsString=__new0  BranchType=R  Resistance=1e6  Inductance=1.0  SetiL0=off  InitialCurrent=0  Capacitance=1.0  Setx0=off  InitialVoltage=0  Measurements=None
  c : powerlib/Elements/Series RLC Branch  LConnTagsString=__new0  RConnTagsString=__new0  BranchType=C  Resistance=1  Inductance=1.0  SetiL0=off  InitialCurrent=0  Capacitance=5e-6  Setx0=off  InitialVoltage=0  Measurements=None
  1 : PMIOPort  Port=1  Side=Left
  2 : PMIOPort  Port=2  Side=Left
  3 : PMIOPort  Port=3  Side=Right
  connections:
  3/RConn1 -- c/RConn1
  1/RConn1 -- R/LConn1 -- L/LConn1
  c/LConn1 -- R/RConn1 -- D/RConn1 -- R1/RConn1
  2/RConn1 -- D/LConn1 -- R1/LConn1 -- L/RConn1

== matlab function SPWM_Mode1/Ton Calc mode1 ==
  data: Ia input double; Ib input double; Ic input double; TonAp output double; TonA23 output double; TonAn output double; TonBp output double; TonB23 output double; Va input double; Vb input double; Vc input double; VdcBalFactor input double; Vdc input double; Ts input double; TonBn output double; TonCp output double; TonC23 output double; TonCn output double; ModulateModeA input double; ModulateModeB input double; ModulateModeC input double
function [TonAp,TonA23,TonAn,TonBp,TonB23,TonBn,TonCp,TonC23,TonCn]  = fcn(Ia,Ib,Ic,Va,Vb,Vc,VdcBalFactor,Vdc,Ts,ModulateModeA,ModulateModeB,ModulateModeC)
%#codegen

%ClarkTrans
Valfa =Va*2/3 - (Vb+Vc)/3;
Vbeta =(Vb-Vc) * sqrt(3)/3;

%调制比计算
m =sqrt(3*(Valfa*Valfa + Vbeta*Vbeta))/Vdc;

%模式切换判断做滞回处理
Mswitchlow = 0.2;
Mswitchhigh =0.25;

ModeswitchEnable =0;    %%%%%避免报错
if m<Mswitchlow; ModeswitchEnable =1;
elseif m>Mswitchhigh; ModeswitchEnable =0;
end

%主扇区判断
if Va>0;signVa=1;else signVa=0;end
if Vb>0;signVb=1;else signVb=0;end
if Vc>0;signVc=1;else signVc=0;end

%电流方向判断
if Ia>=0;SignIa=1;else SignIa=-1;end
if Ib>=0;SignIb=1;else SignIb=-1;end
if Ic>=0;SignIc=1;else SignIc=-1;end

NoTemp = signVa + 2*signVb + 4*signVc;
Transfor =[1 3 2 5 6 4];

if NoTemp ==0; NoTemp =1;
elseif NoTemp ==7; NoTemp =4;
end

MainSectorNo = Transfor(NoTemp);

%零序电压注入母线均衡控制
switch MainSectorNo

    case 1
        VdcBalanceFactorAct = VdcBalFactor*SignIa;

    case 2
        VdcBalanceFactorAct = -VdcBalFactor*SignIc;
        
    case 3
        VdcBalanceFactorAct = VdcBalFactor*SignIb;
        
    case 4
        VdcBalanceFactorAct = -VdcBalFactor*SignIa;
          
    case 5
        VdcBalanceFactorAct = VdcBalFactor*SignIc;
         
    case 6
        VdcBalanceFactorAct = -VdcBalFactor*SignIb;
        
    otherwise
        VdcBalanceFactorAct = -VdcBalFactor*SignIb;
end

%叠加零序提高母线利用率
Vz= max(Va,max(Vb,Vc)) + min(Va,min(Vb,Vc));

Va = Va - Vz/2 -VdcBalanceFactorAct*Vdc/2;
Vb = Vb - Vz/2 -VdcBalanceFactorAct*Vdc/2;
Vc = Vc - Vz/2 -VdcBalanceFactorAct*Vdc/2;

%最小脉宽限制
Tmin  =50e-6;   %最小脉宽限制100us
Tdead =0;        %死区时间64us
TminAct =Tmin+Tdead;

%SPWM发波系数计算
if ModeswitchEnable ==0;
SPWMCoef = 2*Ts/Vdc;
else
SPWMCoef = Ts/Vdc;
end

%三相调制波计算
Taon =Va * SPWMCoef;
Tbon =Vb * SPWMCoef;
Tcon =Vc * SPWMCoef;

%主扇区判断
if Taon>0;signTa=1;else signTa=0;end
if Tbon>0;signTb=1;else signTb=0;end
if Tcon>0;signTc=1;else signTc=0;end

if ModeswitchEnable ==0;
    if ModulateModeA ==0;
    TonAp =Taon; TonAn =Taon +Ts; TonA23 =signTa*Ts;
    else
    TonAp =signTa*Ts; TonAn =signTa*Ts; TonA23 =Taon +(1-signTa)*Ts;
    end

    if ModulateModeB ==0;
    TonBp =Tbon; TonBn =Tbon +Ts; TonB23 =signTb*Ts;
    else
    TonBp =signTb*Ts; TonBn =signTb*Ts; TonB23 =Tbon +(1-signTb)*Ts;
    end

    if ModulateModeC ==0;
    TonCp =Tcon; TonCn =Tcon +Ts; TonC23 =signTc*Ts;
    else
    TonCp =signTc*Ts; TonCn =signTc*Ts; TonC23 =Tcon +(1-signTc)*Ts;
    end  
else
    if ModulateModeA ==0;
    TonAp =Taon + Ts/4; TonAn =Taon +Ts*3/4; TonA23 =Ts/2;
    else
    TonAp =Ts/2; TonAn =Ts/2; TonA23 =2*Taon +Ts/2;
    end

    if ModulateModeB ==0;
    TonBp =Tbon + Ts/4; TonBn =Tbon +Ts*3/4; TonB23 =Ts/2;
    else
    TonBp =Ts/2; TonBn =Ts/2; TonB23 =2*Tbon +Ts/2;
    end

    if ModulateModeC ==0;
    TonCp =Tcon + Ts/4; TonCn =Tcon +Ts*3/4; TonC23 =Ts/2;
    else
    TonCp =Ts/2; TonCn =Ts/2; TonC23 =2*Tcon +Ts/2;
    end  
end 

%小脉宽处理
%A相
if      TonAp<TminAct/2;                              TonAp =0;
elseif  TminAct/2<=TonAp && TonAp<TminAct;            TonAp =TminAct;
elseif  (Ts-TminAct)<=TonAp && TonAp<(Ts-TminAct/2);  TonAp =Ts -TminAct;
elseif  (Ts-TminAct/2)<=TonAp;                        TonAp =Ts;
end

if      TonAn<TminAct/2;                              TonAn =0;
elseif  TminAct/2<=TonAn && TonAn<TminAct;            TonAn =TminAct;
elseif  (Ts-TminAct)<=TonAn && TonAn<(Ts-TminAct/2);  TonAn =Ts -TminAct;
elseif  (Ts-TminAct/2)<=TonAn;                        TonAn =Ts;
end

if      TonA23<TminAct/2;                              TonA23 =0;
elseif  TminAct/2<=TonA23 && TonA23<TminAct;           TonA23 =TminAct;
elseif  (Ts-TminAct)<=TonA23 && TonA23<(Ts-TminAct/2); TonA23 =Ts -TminAct;
elseif  (Ts-TminAct/2)<=TonA23;                        TonA23 =Ts;
end

%B相
if      TonBp<TminAct/2;                              TonBp =0;
elseif  TminAct/2<=TonBp && TonBp<TminAct;            TonBp =TminAct;
elseif  (Ts-TminAct)<=TonBp && TonBp<(Ts-TminAct/2);  TonBp =Ts -TminAct;
elseif  (Ts-TminAct/2)<=TonBp;                        TonBp =Ts;
end

if      TonBn<TminAct/2;                              TonBn =0;
elseif  TminAct/2<=TonBn && TonBn<TminAct;            TonBn =TminAct;
elseif  (Ts-TminAct)<=TonBn && TonBn<(Ts-TminAct/2);  TonBn =Ts -TminAct;
elseif  (Ts-TminAct/2)<=TonBn;                        TonBn =Ts;
end

if      TonB23<TminAct/2;                              TonB23 =0;
elseif  TminAct/2<=TonB23 && TonB23<TminAct;           TonB23 =TminAct;
elseif  (Ts-TminAct)<=TonB23 && TonB23<(Ts-TminAct/2); TonB23 =Ts -TminAct;
elseif  (Ts-TminAct/2)<=TonB23;                        TonB23 =Ts;
end

%C相
if      TonCp<TminAct/2;                              TonCp =0;
elseif  TminAct/2<=TonCp && TonCp<TminAct;            TonCp =TminAct;
elseif  (Ts-TminAct)<=TonCp && TonCp<(Ts-TminAct/2);  TonCp =Ts -TminAct;
elseif  (Ts-TminAct/2)<=TonCp;                        TonCp =Ts;
end

if      TonCn<TminAct/2;                              TonCn =0;
elseif  TminAct/2<=TonCn && TonCn<TminAct;            TonCn =TminAct;
elseif  (Ts-TminAct)<=TonCn && TonCn<(Ts-TminAct/2);  TonCn =Ts -TminAct;
elseif  (Ts-TminAct/2)<=TonCn;                        TonCn =Ts;
end

if      TonC23<TminAct/2;                              TonC23 =0;
elseif  TminAct/2<=TonC23 && TonC23<TminAct;           TonC23 =TminAct;
elseif  (Ts-TminAct)<=TonC23 && TonC23<(Ts-TminAct/2); TonC23 =Ts -TminAct;
elseif  (Ts-TminAct/2)<=TonC23;                        TonC23 =Ts;
end
